simulink model "flightControlSystem"  (R2022b)
settings: Solver=ode3  StartTime=0  StopTime=TFinal  FixedStep=Ts  RelTol=1e-3  EnableMultiTasking=on
undefined symbols (not defined in the file): Ts
libraries: simulink x6
settings Model: ExtModeTrigDuration=80  Creator=The MathWorks, Inc.  LastModifiedBy=The MathWorks, Inc.
settings SolverCC: AlgebraicLoopSolver=TrustRegion
settings DataIOCC: LimitDataPoints=on  SaveFormat=StructureWithTime  ReturnWorkspaceOutputs=off
settings OptimizationCC: BlockReduction=off  BufferReuse=off  PassReuseOutputArgsThreshold=0  MaxStackSize=64
settings DebuggingCC: AlgebraicLoopMsg=none  ParameterPrecisionLossMsg=none  ParameterTunabilityLossMsg=error  BusObjectLabelMismatch=error  SFUnexpectedBacktrackingDiag=warning  SFNoUnconditionalDefaultTransitionDiag=warning  SFExecutionAtInitializationDiag=none  SFMachineParentedDataDiag=warning  ArithmeticOperatorsInVariantConditions=warning
settings HardwareCC: ProdBitPerPointer=32  ProdBitPerSizeT=32  ProdBitPerPtrDiffT=32  ProdLargestAtomicInteger=Long  ProdWordSize=32  ProdHWDeviceType=ARM Compatible->ARM 9  UseEmbeddedCoderFeatures=off  UseSimulinkCoderFeatures=off
settings ModelReferenceCC: EnableRefExpFcnMdlSchedulingChecks=on  ModelReferenceNumInstancesAllowed=Single  PropagateSignalLabelsOutOfModel=off
settings SFSimCC: SimUseLocalCustomCode=off  MATLABDynamicMemAlloc=off  CustomCodeUndefinedFunction=UseInterfaceOnly
settings RTWCC: Description=Embedded Coder  SystemTargetFile=ert.tlc  HardwareBoard=PARROT Mambo  TLCOptions=-aInlineSetEventsForThisBaseRateFcn=TLC_FALSE -aSuppressMultiTaskScheduler=TLC_FALSE -aRateBasedStepFcn=1  TemplateMakefile=ert_default_tmf  GenerateReport=on  RTWUseLocalCustomCode=off  Toolchain=Sourcery G++ Lite GNU Toolchain for Drones  LaunchReport=on
settings CodeAppCC: ForceParamTrailComments=on  MaxIdLength=63  OperatorAnnotations=on
settings ERTTargetCC: ERTCustomFileBanners=off  SupportContinuousTime=on  SupportNonInlinedSFcns=on  RemoveResetFunc=off  ModelStepFunctionPrototypeControlCompliant=off
settings ConfigComp: CovMetricSettings=dw  CovSaveCumulativeToWorkspaceVar=on  CovSaveSingleToWorkspaceVar=on  CovExternalEMLEnable=off  CovSFcnEnable=off

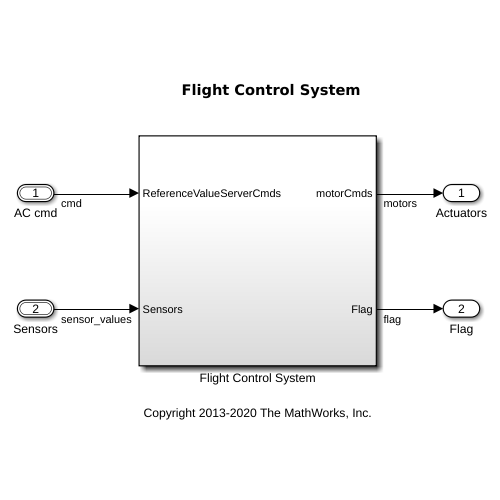
[thumbnail: Simulink's stored preview of the top-level diagram]
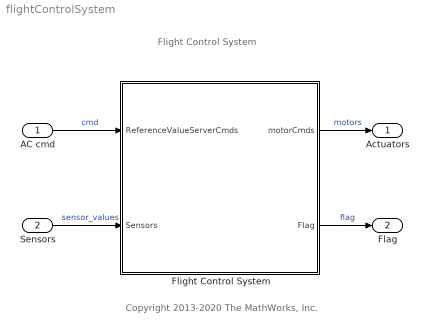
== system flightControlSystem ==
  note: Copyright 2013-2020 The MathWorks, Inc.
  note: Flight Control System
  AC cmd : Inport  OutDataTypeStr=Bus: CommandBus  BusOutputAsStruct=on
  Sensors : Inport  Port=2  OutDataTypeStr=Bus: SensorsBus  BusOutputAsStruct=on
  Flight Control System : Subsystem
  Actuators : Outport  OutDataTypeStr=single  PortDimensions=4  VectorParamsAs1DForOutWhenUnconnected=off
  Flag : Outport  Port=2  OutDataTypeStr=uint8  PortDimensions=1  VectorParamsAs1DForOutWhenUnconnected=off
  wires:
  AC cmd/1 -> Flight Control System/1(ReferenceValueServerCmds)  "cmd"
  Flight Control System/1(motorCmds) -> Actuators/1  "motors"
  Sensors/1 -> Flight Control System/2(Sensors)  "sensor_values"
  Flight Control System/2(Flag) -> Flag/1  "flag"

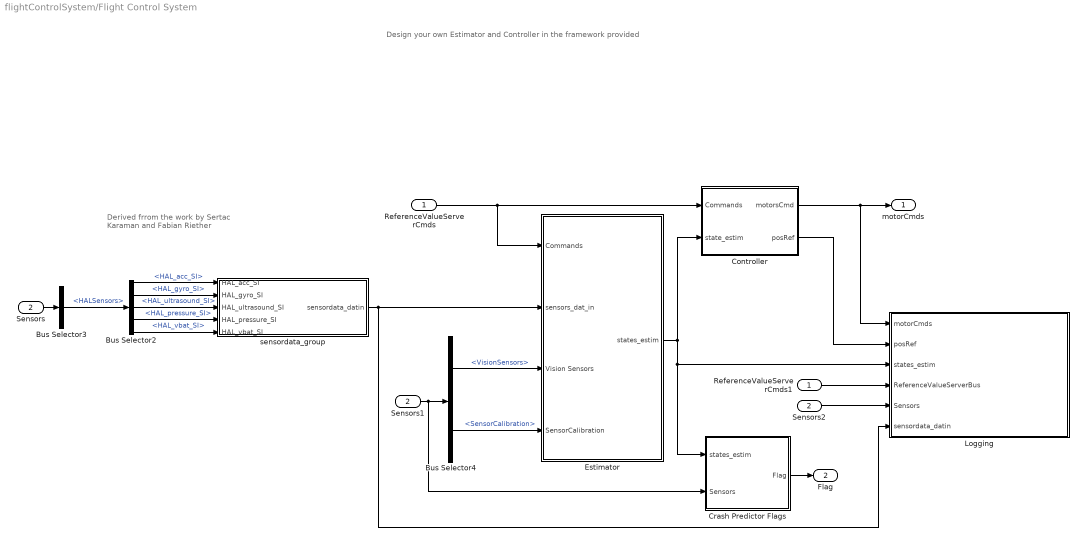
== system flightControlSystem/Flight Control System ==
  note: Derived frrom the work by Sertac
      | Karaman and Fabian Riether
  note: Design your own Estimator and Controller in the framework provided
  ReferenceValueServerCmds : Inport
  Sensors : Inport  Port=2  OutDataTypeStr=Bus: SensorsBus  BusOutputAsStruct=on
  Bus Selector2 : BusSelector  OutputSignals=HAL_acc_SI,HAL_gyro_SI,HAL_ultrasound_SI,HAL_pressure_SI,HAL_vbat_SI
  Bus Selector3 : BusSelector  OutputSignals=HALSensors
  Bus Selector4 : BusSelector  OutputSignals=VisionSensors,SensorCalibration
  Controller : Subsystem
  Crash Predictor Flags : Subsystem
  Estimator : Subsystem
  Logging : Subsystem
      settings: RTWFcnNameOpts=Use subsystem name
  ReferenceValueServerCmds1 : InportShadow
  Sensors1 : InportShadow  Port=2  OutDataTypeStr=Bus: SensorsBus  BusOutputAsStruct=on
  Sensors2 : InportShadow  Port=2  OutDataTypeStr=Bus: SensorsBus  BusOutputAsStruct=on
  sensordata_group : Subsystem
  motorCmds : Outport  VectorParamsAs1DForOutWhenUnconnected=off
  Flag : Outport  Port=2  VectorParamsAs1DForOutWhenUnconnected=off
  wires:
  ReferenceValueServerCmds/1 -> Estimator/1(Commands), Controller/1(Commands)
  Bus Selector2/1 -> sensordata_group/1(HAL_acc_SI)  "<HAL_acc_SI>"
  Bus Selector2/2 -> sensordata_group/2(HAL_gyro_SI)  "<HAL_gyro_SI>"
  Bus Selector2/4 -> sensordata_group/4(HAL_pressure_SI)  "<HAL_pressure_SI>"
  Bus Selector2/3 -> sensordata_group/3(HAL_ultrasound_SI)  "<HAL_ultrasound_SI>"
  Bus Selector4/2 -> Estimator/4(SensorCalibration)  "<SensorCalibration>"
  Estimator/1(states_estim) -> Controller/2(state_estim), Logging/3(states_estim), Crash Predictor Flags/1(states_estim)
  Sensors2/1 -> Logging/5(Sensors)
  Controller/2(posRef) -> Logging/2(posRef)
  ReferenceValueServerCmds1/1 -> Logging/4(ReferenceValueServerBus)
  Controller/1(motorsCmd) -> Logging/1(motorCmds), motorCmds/1
  sensordata_group/1(sensordata_datin) -> Estimator/2(sensors_dat_in), Logging/6(sensordata_datin)
  Bus Selector2/5 -> sensordata_group/5(HAL_vbat_SI)  "<HAL_vbat_SI>"
  Crash Predictor Flags/1(Flag) -> Flag/1
  Sensors1/1 -> Crash Predictor Flags/2(Sensors), Bus Selector4/1
  Sensors/1 -> Bus Selector3/1
  Bus Selector3/1 -> Bus Selector2/1  "<HALSensors>"
  Bus Selector4/1 -> Estimator/3(Vision Sensors)  "<VisionSensors>"

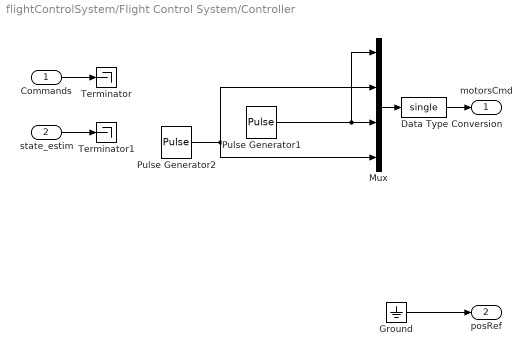
== system flightControlSystem/Flight Control System/Controller ==
  Commands : Inport
  state_estim : Inport  Port=2
  Data Type Conversion : DataTypeConversion  OutDataTypeStr=single  SaturateOnIntegerOverflow=off  RndMeth=Floor
  Ground : Ground
  Mux : Mux
  Pulse Generator1 : DiscretePulseGenerator  Amplitude=400  Period=800  PulseWidth=400  SampleTime=Ts
  Pulse Generator2 : DiscretePulseGenerator  Amplitude=400  Period=800  PulseWidth=400  PhaseDelay=400  SampleTime=Ts
  Terminator : Terminator
  Terminator1 : Terminator
  motorsCmd : Outport  OutDataTypeStr=single  PortDimensions=4  VectorParamsAs1DForOutWhenUnconnected=off
  posRef : Outport  Port=2  VectorParamsAs1DForOutWhenUnconnected=off
  wires:
  Commands/1 -> Terminator/1
  state_estim/1 -> Terminator1/1
  Ground/1 -> posRef/1
  Data Type Conversion/1 -> motorsCmd/1
  Mux/1 -> Data Type Conversion/1
  Pulse Generator1/1 -> Mux/1, Mux/3
  Pulse Generator2/1 -> Mux/2, Mux/4

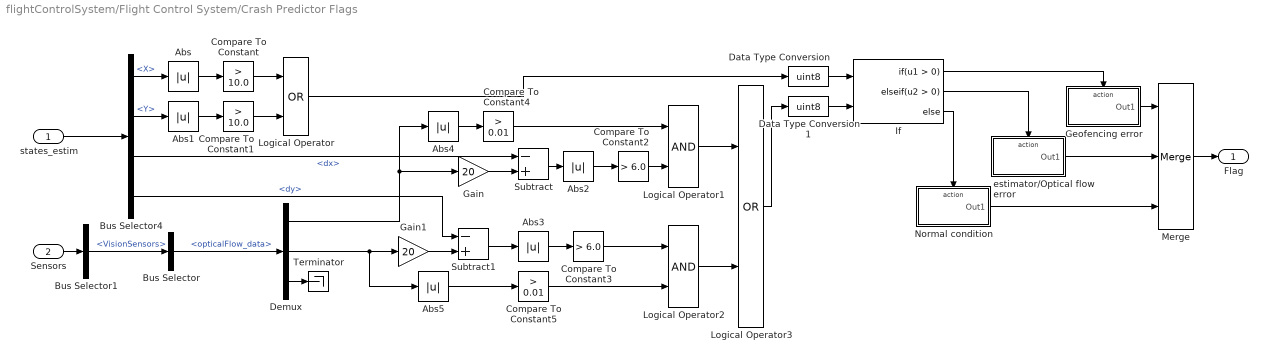
== system flightControlSystem/Flight Control System/Crash Predictor Flags ==
  states_estim : Inport
  Sensors : Inport  Port=2
  Abs{,1..5} (6 alike) : Abs  SaturateOnIntegerOverflow=off
  Bus Selector : BusSelector  OutputSignals=opticalFlow_data
  Bus Selector1 : BusSelector  OutputSignals=VisionSensors
  Bus Selector4 : BusSelector  OutputSignals=X,Y,dx,dy
  Compare To Constant : simulink/Logic and Bit Operations/Compare To Constant  relop=>  const=10.0  OutDataTypeStr=boolean
  Compare To Constant1 : simulink/Logic and Bit Operations/Compare To Constant  relop=>  const=10.0  OutDataTypeStr=boolean
  Compare To Constant2 : simulink/Logic and Bit Operations/Compare To Constant  relop=>  const=6.0  OutDataTypeStr=boolean
  Compare To Constant3 : simulink/Logic and Bit Operations/Compare To Constant  relop=>  const=6.0  OutDataTypeStr=boolean
  Compare To Constant4 : simulink/Logic and Bit Operations/Compare To Constant  relop=>  const=0.01  OutDataTypeStr=boolean
  Compare To Constant5 : simulink/Logic and Bit Operations/Compare To Constant  relop=>  const=0.01  OutDataTypeStr=boolean
  Data Type Conversion : DataTypeConversion  OutDataTypeStr=uint8  RndMeth=Nearest  SaturateOnIntegerOverflow=off
  Data Type Conversion1 : DataTypeConversion  OutDataTypeStr=uint8  RndMeth=Nearest  SaturateOnIntegerOverflow=off
  Demux : Demux  Outputs=3
  Gain : Gain  Gain=20
  Gain1 : Gain  Gain=20
  Geofencing error : Subsystem  TreatAsAtomicUnit=on
  If : If  NumInputs=2  ElseIfExpressions=u2 > 0
  Logical Operator : Logic  Operator=OR  AllPortsSameDT=off
  Logical Operator1 : Logic  AllPortsSameDT=off  OutDataTypeStr=boolean
  Logical Operator2 : Logic  AllPortsSameDT=off  OutDataTypeStr=boolean
  Logical Operator3 : Logic  Operator=OR  AllPortsSameDT=off
  Merge : Merge  Inputs=3  InitialOutput=0
  Normal condition : Subsystem  TreatAsAtomicUnit=on
  Subtract : Sum  Inputs=-+
  Subtract1 : Sum  Inputs=-+
  Terminator : Terminator
  estimator/Optical flow error : Subsystem  TreatAsAtomicUnit=on
  Flag : Outport  VectorParamsAs1DForOutWhenUnconnected=off
  wires:
  Bus Selector4/1 -> Abs/1  "<X>"
  states_estim/1 -> Bus Selector4/1
  Bus Selector4/2 -> Abs1/1  "<Y>"
  Compare To Constant/1 -> Logical Operator/1
  Compare To Constant1/1 -> Logical Operator/2
  Abs/1 -> Compare To Constant/1
  Abs1/1 -> Compare To Constant1/1
  Logical Operator/1 -> Data Type Conversion/1
  Bus Selector/1 -> Demux/1  "<opticalFlow_data>"
  Demux/1 -> Gain/1, Abs4/1
  Demux/2 -> Abs5/1, Gain1/1
  Bus Selector4/3 -> Subtract/1  "<dx>"
  Subtract/1 -> Abs2/1
  Subtract1/1 -> Abs3/1
  Abs2/1 -> Compare To Constant2/1
  Abs3/1 -> Compare To Constant3/1
  Compare To Constant5/1 -> Logical Operator2/2
  Abs4/1 -> Compare To Constant4/1
  Abs5/1 -> Compare To Constant5/1
  Compare To Constant3/1 -> Logical Operator2/1
  Logical Operator1/1 -> Logical Operator3/1
  Logical Operator2/1 -> Logical Operator3/2
  Logical Operator3/1 -> Data Type Conversion1/1
  Demux/3 -> Terminator/1
  Gain/1 -> Subtract/2
  Bus Selector4/4 -> Subtract1/1  "<dy>"
  Gain1/1 -> Subtract1/2
  Compare To Constant4/1 -> Logical Operator1/1
  Compare To Constant2/1 -> Logical Operator1/2
  Sensors/1 -> Bus Selector1/1
  Bus Selector1/1 -> Bus Selector/1  "<VisionSensors>"
  Merge/1 -> Flag/1
  If/1 -> Geofencing error/Action
  If/2 -> estimator/Optical flow error/Action
  If/3 -> Normal condition/Action
  Geofencing error/1(Out1) -> Merge/1
  estimator/Optical flow error/1(Out1) -> Merge/2
  Normal condition/1(Out1) -> Merge/3
  Data Type Conversion/1 -> If/1
  Data Type Conversion1/1 -> If/2

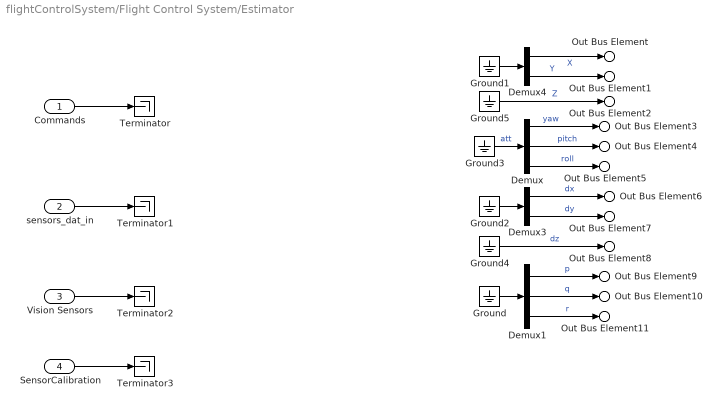
== system flightControlSystem/Flight Control System/Estimator ==
  Commands : Inport
  sensors_dat_in : Inport  Port=2
  Vision Sensors : Inport  Port=3
  SensorCalibration : Inport  Port=4
  Demux : Demux  Outputs=3
  Demux1 : Demux  Outputs=3
  Demux3 : Demux  Outputs=2
  Demux4 : Demux  Outputs=2
  Ground{,1..5} (6 alike) : Ground
  Terminator{,1..3} (4 alike) : Terminator
  Out Bus Element : Outport  VectorParamsAs1DForOutWhenUnconnected=off  PortName=states_estim  Element=X
  Out Bus Element1 : Outport  VectorParamsAs1DForOutWhenUnconnected=off  PortName=states_estim  Element=Y
  Out Bus Element2 : Outport  VectorParamsAs1DForOutWhenUnconnected=off  PortName=states_estim  Element=Z
  Out Bus Element3 : Outport  VectorParamsAs1DForOutWhenUnconnected=off  PortName=states_estim  Element=yaw
  Out Bus Element4 : Outport  VectorParamsAs1DForOutWhenUnconnected=off  PortName=states_estim  Element=pitch
  Out Bus Element5 : Outport  VectorParamsAs1DForOutWhenUnconnected=off  PortName=states_estim  Element=roll
  Out Bus Element6 : Outport  VectorParamsAs1DForOutWhenUnconnected=off  PortName=states_estim  Element=dx
  Out Bus Element7 : Outport  VectorParamsAs1DForOutWhenUnconnected=off  PortName=states_estim  Element=dy
  Out Bus Element8 : Outport  VectorParamsAs1DForOutWhenUnconnected=off  PortName=states_estim  Element=dz
  Out Bus Element9 : Outport  VectorParamsAs1DForOutWhenUnconnected=off  PortName=states_estim  Element=p
  Out Bus Element10 : Outport  VectorParamsAs1DForOutWhenUnconnected=off  PortName=states_estim  Element=q
  Out Bus Element11 : Outport  VectorParamsAs1DForOutWhenUnconnected=off  PortName=states_estim  Element=r
  wires:
  Ground5/1 -> Out Bus Element2/1  "Z"
  Demux/2 -> Out Bus Element4/1  "pitch"
  Demux4/1 -> Out Bus Element/1  "X"
  Demux3/1 -> Out Bus Element6/1  "dx"
  Ground4/1 -> Out Bus Element8/1  "dz"
  Demux/1 -> Out Bus Element3/1  "yaw"
  Demux1/1 -> Out Bus Element9/1  "p"
  Demux4/2 -> Out Bus Element1/1  "Y"
  Ground1/1 -> Demux4/1
  Ground2/1 -> Demux3/1
  Demux/3 -> Out Bus Element5/1  "roll"
  Ground3/1 -> Demux/1  "att"
  Demux1/2 -> Out Bus Element10/1  "q"
  Demux1/3 -> Out Bus Element11/1  "r"
  Demux3/2 -> Out Bus Element7/1  "dy"
  Ground/1 -> Demux1/1
  Commands/1 -> Terminator/1
  sensors_dat_in/1 -> Terminator1/1
  SensorCalibration/1 -> Terminator3/1
  Vision Sensors/1 -> Terminator2/1

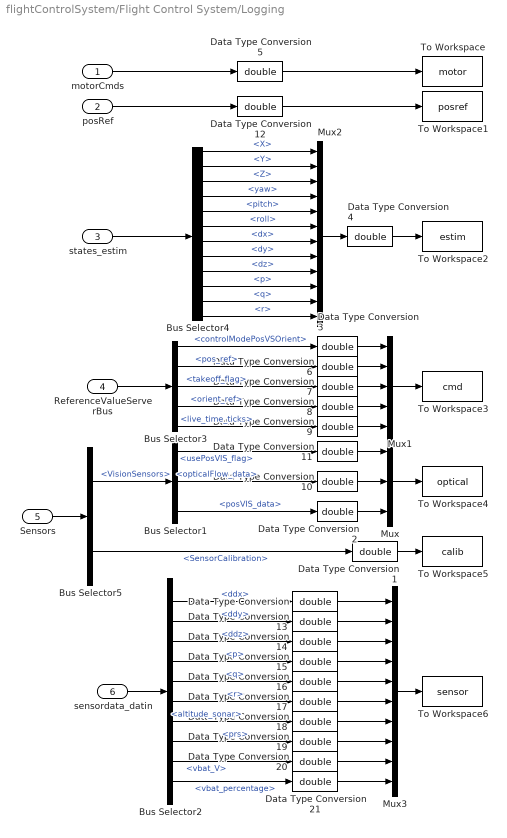
== system flightControlSystem/Flight Control System/Logging ==
  motorCmds : Inport
  posRef : Inport  Port=2
  states_estim : Inport  Port=3  OutDataTypeStr=Bus: statesEstim_t  BusOutputAsStruct=on
  ReferenceValueServerBus : Inport  Port=4  OutDataTypeStr=Bus: CommandBus  BusOutputAsStruct=on
  Sensors : Inport  Port=5  OutDataTypeStr=Bus: SensorsBus
  sensordata_datin : Inport  Port=6  OutDataTypeStr=Bus: sensordata_t
  Bus Selector1 : BusSelector  OutputSignals=usePosVIS_flag,opticalFlow_data,posVIS_data
  Bus Selector2 : BusSelector  OutputSignals=ddx,ddy,ddz,p,q,r,altitude_sonar,prs,vbat_V,vbat_percentage
  Bus Selector3 : BusSelector  OutputSignals=controlModePosVSOrient,pos_ref,takeoff_flag,orient_ref,live_time_ticks
  Bus Selector4 : BusSelector  OutputSignals=X,Y,Z,yaw,pitch,roll,dx,dy,dz,p,q,r
  Bus Selector5 : BusSelector  OutputSignals=VisionSensors,SensorCalibration
  Data Type Conversion{,1..21} (22 alike) : DataTypeConversion  OutDataTypeStr=double  SaturateOnIntegerOverflow=off  RndMeth=Floor
  Mux : Mux  Inputs=3
  Mux1 : Mux  Inputs=5
  Mux2 : Mux  Inputs=12
  Mux3 : Mux  Inputs=10
  To Workspace : ToWorkspace  VariableName=motor  SaveFormat=Structure With Time  SampleTime=-1
  To Workspace1 : ToWorkspace  VariableName=posref  SaveFormat=Structure With Time  SampleTime=-1
  To Workspace2 : ToWorkspace  VariableName=estim  SaveFormat=Structure With Time  SampleTime=-1
  To Workspace3 : ToWorkspace  VariableName=cmd  SaveFormat=Structure With Time  SampleTime=-1
  To Workspace4 : ToWorkspace  VariableName=optical  SaveFormat=Structure With Time  SampleTime=-1
  To Workspace5 : ToWorkspace  VariableName=calib  SaveFormat=Structure With Time  SampleTime=-1
  To Workspace6 : ToWorkspace  VariableName=sensor  SaveFormat=Structure With Time  SampleTime=-1
  wires:
  Bus Selector3/1 -> Data Type Conversion3/1  "<controlModePosVSOrient>"
  Bus Selector3/3 -> Data Type Conversion7/1  "<takeoff_flag>"
  Bus Selector3/4 -> Data Type Conversion8/1  "<orient_ref>"
  Bus Selector3/5 -> Data Type Conversion9/1  "<live_time_ticks>"
  ReferenceValueServerBus/1 -> Bus Selector3/1
  Bus Selector3/2 -> Data Type Conversion6/1  "<pos_ref>"
  sensordata_datin/1 -> Bus Selector2/1
  Bus Selector2/1 -> Data Type Conversion/1  "<ddx>"
  Sensors/1 -> Bus Selector5/1
  Bus Selector1/1 -> Data Type Conversion11/1  "<usePosVIS_flag>"
  Bus Selector1/2 -> Data Type Conversion10/1  "<opticalFlow_data>"
  Bus Selector1/3 -> Data Type Conversion2/1  "<posVIS_data>"
  Data Type Conversion1/1 -> To Workspace5/1
  Bus Selector5/2 -> Data Type Conversion1/1  "<SensorCalibration>"
  Mux/1 -> To Workspace4/1
  Data Type Conversion4/1 -> To Workspace2/1
  motorCmds/1 -> Data Type Conversion5/1
  Data Type Conversion5/1 -> To Workspace/1
  Mux1/1 -> To Workspace3/1
  states_estim/1 -> Bus Selector4/1
  Mux2/1 -> Data Type Conversion4/1
  Bus Selector4/4 -> Mux2/4  "<yaw>"
  Bus Selector4/6 -> Mux2/6  "<roll>"
  Bus Selector4/5 -> Mux2/5  "<pitch>"
  Bus Selector4/9 -> Mux2/9  "<dz>"
  Bus Selector4/7 -> Mux2/7  "<dx>"
  Bus Selector4/8 -> Mux2/8  "<dy>"
  Bus Selector4/10 -> Mux2/10  "<p>"
  Bus Selector4/12 -> Mux2/12  "<r>"
  Bus Selector4/2 -> Mux2/2  "<Y>"
  Bus Selector4/11 -> Mux2/11  "<q>"
  Bus Selector4/3 -> Mux2/3  "<Z>"
  Bus Selector4/1 -> Mux2/1  "<X>"
  Data Type Conversion3/1 -> Mux1/1
  Data Type Conversion6/1 -> Mux1/2
  Data Type Conversion7/1 -> Mux1/3
  Data Type Conversion8/1 -> Mux1/4
  Data Type Conversion9/1 -> Mux1/5
  Data Type Conversion2/1 -> Mux/3
  Data Type Conversion10/1 -> Mux/2
  Data Type Conversion11/1 -> Mux/1
  posRef/1 -> Data Type Conversion12/1
  Data Type Conversion12/1 -> To Workspace1/1
  Bus Selector2/2 -> Data Type Conversion13/1  "<ddy>"
  Bus Selector2/3 -> Data Type Conversion14/1  "<ddz>"
  Bus Selector2/4 -> Data Type Conversion15/1  "<p>"
  Bus Selector2/5 -> Data Type Conversion16/1  "<q>"
  Bus Selector2/6 -> Data Type Conversion17/1  "<r>"
  Bus Selector2/7 -> Data Type Conversion18/1  "<altitude_sonar>"
  Bus Selector2/8 -> Data Type Conversion19/1  "<prs>"
  Bus Selector2/9 -> Data Type Conversion20/1  "<vbat_V>"
  Bus Selector2/10 -> Data Type Conversion21/1  "<vbat_percentage>"
  Data Type Conversion/1 -> Mux3/1
  Data Type Conversion13/1 -> Mux3/2
  Data Type Conversion14/1 -> Mux3/3
  Data Type Conversion15/1 -> Mux3/4
  Data Type Conversion16/1 -> Mux3/5
  Data Type Conversion17/1 -> Mux3/6
  Data Type Conversion18/1 -> Mux3/7
  Data Type Conversion19/1 -> Mux3/8
  Data Type Conversion20/1 -> Mux3/9
  Data Type Conversion21/1 -> Mux3/10
  Mux3/1 -> To Workspace6/1
  Bus Selector5/1 -> Bus Selector1/1  "<VisionSensors>"

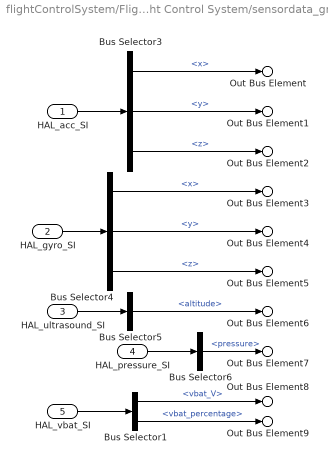
== system flightControlSystem/Flight Control System/sensordata_group ==
  HAL_acc_SI : Inport  OutDataTypeStr=Bus: HAL_acc_SI_t
  HAL_gyro_SI : Inport  Port=2  OutDataTypeStr=Bus: HAL_gyro_SI_t
  HAL_ultrasound_SI : Inport  Port=3  OutDataTypeStr=Bus: HAL_ultrasound_SI_t
  HAL_pressure_SI : Inport  Port=4  OutDataTypeStr=Bus: HAL_pressure_SI_t
  HAL_vbat_SI : Inport  Port=5  OutDataTypeStr=Bus: HAL_vbat_SI_t
  Bus Selector1 : BusSelector  OutputSignals=vbat_V,vbat_percentage
  Bus Selector3 : BusSelector  OutputSignals=x,y,z
  Bus Selector4 : BusSelector  OutputSignals=x,y,z
  Bus Selector5 : BusSelector  OutputSignals=altitude
  Bus Selector6 : BusSelector  OutputSignals=pressure
  Out Bus Element : Outport  VectorParamsAs1DForOutWhenUnconnected=off  PortName=sensordata_datin  Element=ddx
  Out Bus Element1 : Outport  VectorParamsAs1DForOutWhenUnconnected=off  PortName=sensordata_datin  Element=ddy
  Out Bus Element2 : Outport  VectorParamsAs1DForOutWhenUnconnected=off  PortName=sensordata_datin  Element=ddz
  Out Bus Element3 : Outport  VectorParamsAs1DForOutWhenUnconnected=off  PortName=sensordata_datin  Element=p
  Out Bus Element4 : Outport  VectorParamsAs1DForOutWhenUnconnected=off  PortName=sensordata_datin  Element=q
  Out Bus Element5 : Outport  VectorParamsAs1DForOutWhenUnconnected=off  PortName=sensordata_datin  Element=r
  Out Bus Element6 : Outport  VectorParamsAs1DForOutWhenUnconnected=off  PortName=sensordata_datin  Element=altitude_sonar
  Out Bus Element7 : Outport  VectorParamsAs1DForOutWhenUnconnected=off  PortName=sensordata_datin  Element=prs
  Out Bus Element8 : Outport  VectorParamsAs1DForOutWhenUnconnected=off  PortName=sensordata_datin  Element=vbat_V
  Out Bus Element9 : Outport  VectorParamsAs1DForOutWhenUnconnected=off  PortName=sensordata_datin  Element=vbat_percentage
  wires:
  HAL_gyro_SI/1 -> Bus Selector4/1
  HAL_acc_SI/1 -> Bus Selector3/1
  HAL_pressure_SI/1 -> Bus Selector6/1
  HAL_ultrasound_SI/1 -> Bus Selector5/1
  Bus Selector4/1 -> Out Bus Element3/1  "<x>"
  Bus Selector3/3 -> Out Bus Element2/1  "<z>"
  Bus Selector4/3 -> Out Bus Element5/1  "<z>"
  Bus Selector5/1 -> Out Bus Element6/1  "<altitude>"
  Bus Selector6/1 -> Out Bus Element7/1  "<pressure>"
  Bus Selector4/2 -> Out Bus Element4/1  "<y>"
  Bus Selector3/1 -> Out Bus Element/1  "<x>"
  Bus Selector3/2 -> Out Bus Element1/1  "<y>"
  Bus Selector1/1 -> Out Bus Element8/1  "<vbat_V>"
  HAL_vbat_SI/1 -> Bus Selector1/1
  Bus Selector1/2 -> Out Bus Element9/1  "<vbat_percentage>"

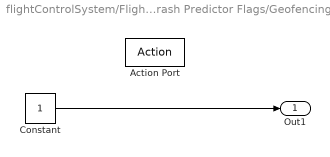
== system flightControlSystem/Flight Control System/Crash Predictor Flags/Geofencing error ==
  Action Port : ActionPort  ActionPortLabel=if { }
  Constant : Constant  OutDataTypeStr=uint8
  Out1 : Outport  VectorParamsAs1DForOutWhenUnconnected=off
  wires:
  Constant/1 -> Out1/1

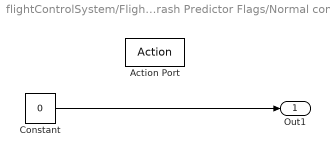
== system flightControlSystem/Flight Control System/Crash Predictor Flags/Normal condition ==
  Action Port : ActionPort  ActionPortLabel=else { }
  Constant : Constant  Value=0  OutDataTypeStr=uint8
  Out1 : Outport  VectorParamsAs1DForOutWhenUnconnected=off
  wires:
  Constant/1 -> Out1/1

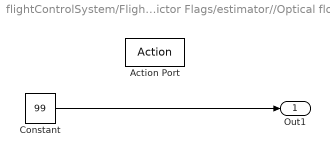
== system flightControlSystem/Flight Control System/Crash Predictor Flags/estimator//Optical flow error ==
  Action Port : ActionPort  ActionPortLabel=elseif { }
  Constant : Constant  Value=99  OutDataTypeStr=uint8
  Out1 : Outport  VectorParamsAs1DForOutWhenUnconnected=off
  wires:
  Constant/1 -> Out1/1
